simulink model "regen_enabled"  (R2023b)
settings: Solver=VariableStepAuto  StartTime=0.0  StopTime=10.0  RelTol=1e-3
settings Model: Creator=no  LastModifiedBy=no

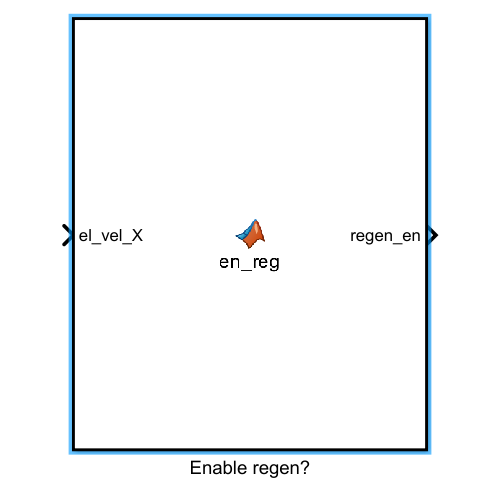
[thumbnail: Simulink's stored preview of the top-level diagram]
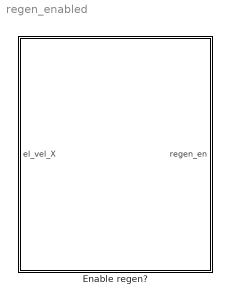
== system regen_enabled ==
  Enable regen? : MATLAB Function  TreatAsAtomicUnit=on

== matlab function regen_enabled/Enable regen? ==
  data: el_vel_X input; regen_en output
function regen_en  = en_reg(el_vel_X)
